simulink model "model"  (R2015a)
settings: Solver=ode45  StartTime=0.0  StopTime=10.0  RelTol=1e-3
settings Model: Creator=Diddharth Singh  LastModifiedBy=Diddharth Singh

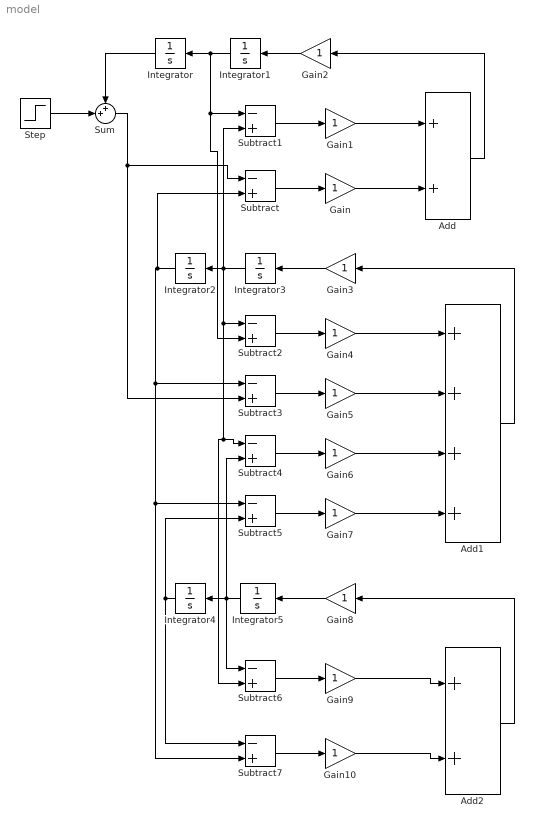
== system model ==
  Add : Sum
  Add1 : Sum  Inputs=++++
  Add2 : Sum
  Gain{,1..10} (11 alike) : Gain
  Integrator{,1..5} (6 alike) : Integrator
  Step : Step  SampleTime=0
  Subtract{,1..7} (8 alike) : Sum  Inputs=-+
  Sum : Sum  Inputs=++|
  wires:
  Subtract/1 -> Gain/1
  Subtract1/1 -> Gain1/1
  Gain1/1 -> Add/1
  Gain/1 -> Add/2
  Add/1 -> Gain2/1
  Gain2/1 -> Integrator1/1
  Integrator1/1 -> Subtract2/2, Subtract1/1, Integrator/1
  Integrator2/1 -> Subtract/2, Subtract7/2, Subtract5/1, Subtract3/1
  Integrator3/1 -> Subtract2/1, Subtract6/2, Subtract4/1, Subtract1/2, Integrator2/1
  Gain3/1 -> Integrator3/1
  Subtract2/1 -> Gain4/1
  Subtract3/1 -> Gain5/1
  Subtract4/1 -> Gain6/1
  Subtract5/1 -> Gain7/1
  Gain7/1 -> Add1/4
  Gain6/1 -> Add1/3
  Gain5/1 -> Add1/2
  Gain4/1 -> Add1/1
  Add1/1 -> Gain3/1
  Integrator4/1 -> Subtract5/2, Subtract7/1
  Integrator5/1 -> Subtract6/1, Subtract4/2, Integrator4/1
  Gain8/1 -> Integrator5/1
  Subtract6/1 -> Gain9/1
  Subtract7/1 -> Gain10/1
  Gain9/1 -> Add2/1
  Gain10/1 -> Add2/2
  Add2/1 -> Gain8/1
  Integrator/1 -> Sum/1
  Sum/1 -> Subtract3/2, Subtract/1
  Step/1 -> Sum/2
